simulink model "enginecontroller"  (R2015a)
settings: Solver=ode45  StartTime=0.0  StopTime=10.0  RelTol=1e-3
undefined symbols (not defined in the file): drive_block, drive_enginemodel, FuelConsTable, GasEmisTable, h, km, s, speed, torque
libraries: driveline x4, aerolibconvert2 x1, simulink x1
settings Model: Creator=Elena  LastModifiedBy=Elena

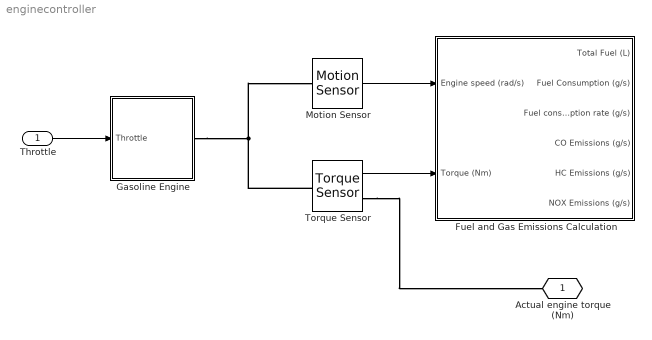
== system enginecontroller ==
  Throttle : Inport
  Fuel and Gas Emissions Calculation : Subsystem
  Gasoline Engine : Subsystem  AncestorBlock=driveline/Vehicle Components/Gasoline Engine  DialogController=PMDialogs.PMDefaultMaskDlg  LoadFcn=drive_block('LoadFcn');  StartFcn=drive_enginemodel('Start');  mask(Gasoline Engine){power_max=57000, speed_at_power_max=5000, speed_max=6000}
      mask prompts: power_max "Maximum power [W]:"; speed_at_power_max "Speed at maximum power [rpm]:"; speed_max "Maximum speed [rpm]:"
      mask help:
      | Simple gasoline fuel engine model with speed governor.  The throttle input signal lies between zero and one and specifies the torque demanded from the engine as a fraction of the maximum possible torque.  This signal also indirectly controls the engine speed.  The engine model does not include air-fuel combustion dynamics.
      |
      | If the throttle signal rises above one or falls below zero, the engine limits the signal to one or zero, respectively. If the engine speed rises above the maximum speed, the engine torque drops to zero.
      mask init:
      | drive_preinitmask();[speed,power,torque,p] = ...
      | 	drive_enginemodel('MaskGasoline');
      settings: CopyFcn=drive_block('CopyFcn');  DeleteFcn=drive_block('DeleteFcn');  ModelCloseFcn=drive_block('ModelCloseFcn');  PreSaveFcn=drive_block('PreSaveFcn');  PostSaveFcn=drive_block('PostSaveFcn');  PreCopyFcn=drive_block('PreCopyFcn');  PreDeleteFcn=drive_block('PreDeleteFcn');
      mask Help: web(drive_help);
      mask Display:
      | image(imread('engine.bmp'),'center')
      | plot(speed, torque/max(torque))
      | plot(speed, power/max(power))
      | port_label('input', 1, 'Throttle')
  Motion Sensor : driveline/Sensors & Actuators/Motion Sensor  Angle=off  x0=0  Velocity=on  Acceleration=off
  Torque Sensor : driveline/Sensors & Actuators/Torque Sensor
  Actual engine torque (Nm) : PMIOPort  Port=1  Side=Left
  wires:
  Throttle/1 -> Gasoline Engine/1(Throttle)
  Motion Sensor/1 -> Fuel and Gas Emissions Calculation/1(Engine speed (rad/s))
  Torque Sensor/1 -> Fuel and Gas Emissions Calculation/2(Torque (Nm))
  connections:
  Torque Sensor/RConn1 -- Actual engine torque (Nm)/RConn1
  Gasoline Engine/RConn1 -- Torque Sensor/LConn1 -- Motion Sensor/LConn1

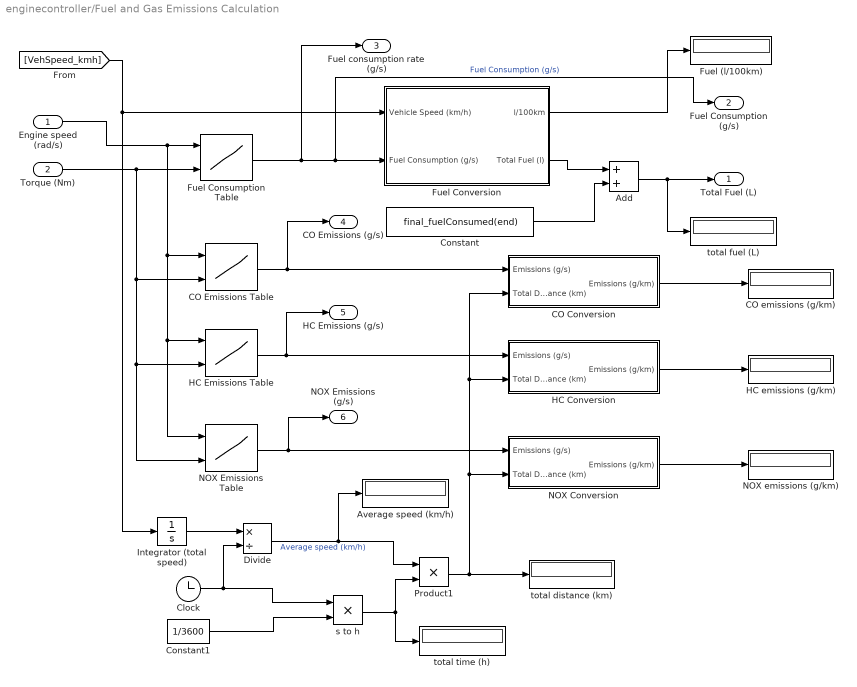
== system enginecontroller/Fuel and Gas Emissions Calculation ==
  Engine speed (rad/s) : Inport
  Torque (Nm) : Inport  Port=2
  Add : Sum
  Average speed (km/h) : Display
      settings: Decimation=100
  CO Conversion : Subsystem
  CO Emissions Table : Lookup2D  RowIndex=GasEmisTable.speed  ColumnIndex=GasEmisTable.torque  Table=GasEmisTable.lookupTableCO  LookUpMeth=Interpolation-Use End Values
  CO emissions (g/km) : Display
      settings: Decimation=100
  Clock : Clock
  Constant : Constant  Value=final_fuelConsumed(end)
  Constant1 : Constant  Value=1/3600
  Divide : Product  Inputs=*/
  Fuel Consumption Table : Lookup2D  RowIndex=FuelConsTable.speed  ColumnIndex=FuelConsTable.torque  Table=FuelConsTable.lookupTableFuel  LookUpMeth=Interpolation-Use End Values
  Fuel (l/100km) : Display
      settings: Decimation=100
  Fuel Conversion : Subsystem
  HC Conversion : Subsystem
  HC Emissions Table : Lookup2D  RowIndex=GasEmisTable.speed  ColumnIndex=GasEmisTable.torque  Table=GasEmisTable.lookupTableHC  LookUpMeth=Interpolation-Use End Values
  HC emissions (g/km) : Display
      settings: Decimation=100
  Integrator (total speed) : Integrator
  NOX Conversion : Subsystem
  NOX Emissions Table : Lookup2D  RowIndex=GasEmisTable.speed  ColumnIndex=GasEmisTable.torque  Table=GasEmisTable.lookupTableNOX  LookUpMeth=Interpolation-Use End Values
  NOX emissions (g/km) : Display
      settings: Decimation=100
  Product1 : Product
  s to h : Product
  total distance (km) : Display
      settings: Decimation=100
  total fuel (L) : Display
      settings: Decimation=100
  total time (h) : Display
      settings: Decimation=100
  Total Fuel (L) : Outport
  Fuel Consumption (g/s) : Outport  Port=2
  Fuel consumption rate (g/s) : Outport  Port=3
  CO Emissions (g/s) : Outport  Port=4
  HC Emissions (g/s) : Outport  Port=5
  NOX Emissions (g/s) : Outport  Port=6
  wires:
  Fuel Conversion/2(Total Fuel (l)) -> Add/1
  Fuel Consumption Table/1 -> Fuel consumption rate (g/s)/1, Fuel Consumption (g/s)/1, Fuel Conversion/2(Fuel Consumption (g/s))  "Fuel Consumption (g/s)"
  Fuel Conversion/1(l/100km) -> Fuel (l/100km)/1
  [VehSpeed_kmh] -> Fuel Conversion/1(Vehicle Speed (km/h)), Integrator (total speed)/1
  Torque (Nm)/1 -> Fuel Consumption Table/2, CO Emissions Table/2, HC Emissions Table/2, NOX Emissions Table/2
  Engine speed (rad/s)/1 -> Fuel Consumption Table/1, NOX Emissions Table/1, HC Emissions Table/1, CO Emissions Table/1
  HC Emissions Table/1 -> HC Conversion/1(Emissions (g/s)), HC Emissions (g/s)/1
  NOX Emissions Table/1 -> NOX Conversion/1(Emissions (g/s)), NOX Emissions (g/s)/1
  CO Emissions Table/1 -> CO Emissions (g/s)/1, CO Conversion/1(Emissions (g/s))
  Constant/1 -> Add/2
  Add/1 -> Total Fuel (L)/1, total fuel (L)/1
  Clock/1 -> s to h/1, Divide/2
  Constant1/1 -> s to h/2
  s to h/1 -> total time (h)/1, Product1/2
  Product1/1 -> NOX Conversion/2(Total Distance (km)), HC Conversion/2(Total Distance (km)), CO Conversion/2(Total Distance (km)), total distance (km)/1
  CO Conversion/1(Emissions (g/km)) -> CO emissions (g/km)/1
  HC Conversion/1(Emissions (g/km)) -> HC emissions (g/km)/1
  NOX Conversion/1(Emissions (g/km)) -> NOX emissions (g/km)/1
  Integrator (total speed)/1 -> Divide/1
  Divide/1 -> Average speed (km/h)/1, Product1/1  "Average speed (km/h)"

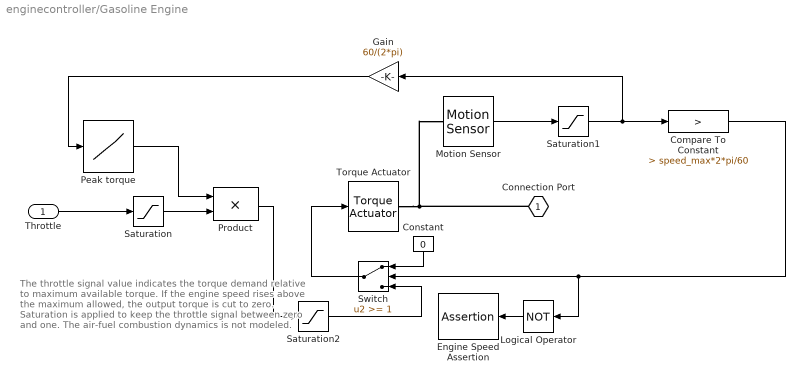
== system enginecontroller/Gasoline Engine ==
  note: The throttle signal value indicates the torque demand
      | relative to maximum available torque. If the engine
      | speed rises above the maximum allowed, the output
      | torque is cut to zero. Saturation is applied to keep the
      | throttle signal between zero and one.
      |
      | The air-fuel combustion dynamics is not modeled.
  Throttle : Inport
  Compare To Constant : simulink/Logic and Bit Operations/Compare To Constant  relop=>  const=speed_max*2*pi/60  OutDataTypeStr=uint8  ZeroCross=off
  Constant : Constant  Value=0
  Engine Speed Assertion : Assertion  AssertionFailFcn=disp('Engine speed (rpm) exceeded maximum speed during the simulation. Simulation results could be inaccurate or unpredictable.')  StopWhenAssertionFail=off
  Gain : Gain  Gain=60/(2*pi)
  Logical Operator : Logic  Operator=NOT  AllPortsSameDT=off  OutDataTypeStr=boolean
  Motion Sensor : driveline/Sensors & Actuators/Motion Sensor  Angle=off  x0=5  Velocity=on  Acceleration=off
  Peak torque : Lookup  InputValues=speed  Table=torque  SaturateOnIntegerOverflow=on
  Product : Product  SaturateOnIntegerOverflow=on  OutDataTypeStr=Inherit: Same as first input
  Saturation : Saturate  UpperLimit=1.0  LowerLimit=0.0
  Saturation1 : Saturate  UpperLimit=6000*pi/30  LowerLimit=0.0
  Saturation2 : Saturate  UpperLimit=136.0757  LowerLimit=0
  Switch : Switch  Threshold=1
  Torque Actuator : driveline/Sensors & Actuators/Torque Actuator
  Connection Port : PMIOPort  Port=1  Side=Right
  wires:
  Saturation/1 -> Product/2
  Throttle/1 -> Saturation/1
  Constant/1 -> Switch/1
  Compare To Constant/1 -> Switch/2, Logical Operator/1
  Product/1 -> Saturation2/1
  Motion Sensor/1 -> Saturation1/1
  Peak torque/1 -> Product/1
  Logical Operator/1 -> Engine Speed Assertion/1
  Saturation1/1 -> Gain/1, Compare To Constant/1
  Switch/1 -> Torque Actuator/1
  Gain/1 -> Peak torque/1
  Saturation2/1 -> Switch/3
  connections:
  Connection Port/RConn1 -- Torque Actuator/RConn1 -- Motion Sensor/LConn1

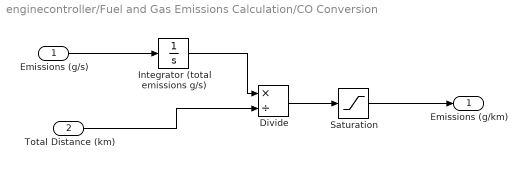
== system enginecontroller/Fuel and Gas Emissions Calculation/CO Conversion ==
  Emissions (g/s) : Inport
  Total Distance (km) : Inport  Port=2
  Divide : Product  Inputs=*/
  Integrator (total emissions g/s) : Integrator  InitialCondition=eps
  Saturation : Saturate  UpperLimit=Inf  LowerLimit=0
  Emissions (g/km) : Outport
  wires:
  Divide/1 -> Saturation/1
  Emissions (g/s)/1 -> Integrator (total emissions g/s)/1
  Integrator (total emissions g/s)/1 -> Divide/1
  Total Distance (km)/1 -> Divide/2
  Saturation/1 -> Emissions (g/km)/1

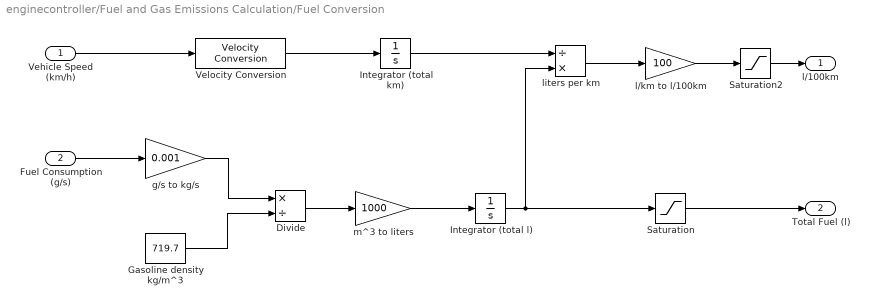
== system enginecontroller/Fuel and Gas Emissions Calculation/Fuel Conversion ==
  Vehicle Speed (km/h) : Inport
  Fuel Consumption (g/s) : Inport  Port=2
  Divide : Product  Inputs=*/
  Gasoline density kg/m^3 : Constant  Value=719.7
  Integrator (total km) : Integrator  InitialCondition=eps
  Integrator (total l) : Integrator  InitialCondition=eps
  Saturation : Saturate  UpperLimit=Inf  LowerLimit=0
  Saturation2 : Saturate  UpperLimit=15  LowerLimit=0
  Velocity Conversion : aerolibconvert2/Velocity Conversion  IU=km/h  OU=km/s
  g/s to kg/s : Gain  Gain=0.001
  l/km to l/100km : Gain  Gain=100
  liters per km : Product  Inputs=/*
  m^3 to liters : Gain  Gain=1000
  l/100km : Outport
  Total Fuel (l) : Outport  Port=2
  wires:
  Vehicle Speed (km/h)/1 -> Velocity Conversion/1
  Velocity Conversion/1 -> Integrator (total km)/1
  Fuel Consumption (g/s)/1 -> g/s to kg/s/1
  g/s to kg/s/1 -> Divide/1
  Gasoline density kg/m^3/1 -> Divide/2
  Divide/1 -> m^3 to liters/1
  m^3 to liters/1 -> Integrator (total l)/1
  Integrator (total km)/1 -> liters per km/1
  Integrator (total l)/1 -> Saturation/1, liters per km/2
  liters per km/1 -> l/km to l/100km/1
  l/km to l/100km/1 -> Saturation2/1
  Saturation/1 -> Total Fuel (l)/1
  Saturation2/1 -> l/100km/1

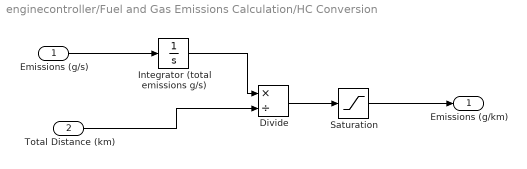
== system enginecontroller/Fuel and Gas Emissions Calculation/HC Conversion ==
  Emissions (g/s) : Inport
  Total Distance (km) : Inport  Port=2
  Divide : Product  Inputs=*/
  Integrator (total emissions g/s) : Integrator  InitialCondition=eps
  Saturation : Saturate  UpperLimit=Inf  LowerLimit=0
  Emissions (g/km) : Outport
  wires:
  Divide/1 -> Saturation/1
  Emissions (g/s)/1 -> Integrator (total emissions g/s)/1
  Integrator (total emissions g/s)/1 -> Divide/1
  Total Distance (km)/1 -> Divide/2
  Saturation/1 -> Emissions (g/km)/1

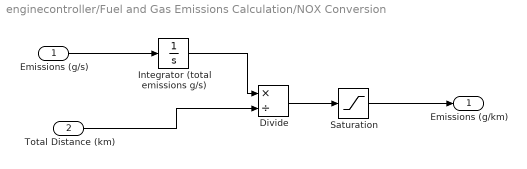
== system enginecontroller/Fuel and Gas Emissions Calculation/NOX Conversion ==
  Emissions (g/s) : Inport
  Total Distance (km) : Inport  Port=2
  Divide : Product  Inputs=*/
  Integrator (total emissions g/s) : Integrator  InitialCondition=eps
  Saturation : Saturate  UpperLimit=Inf  LowerLimit=0
  Emissions (g/km) : Outport
  wires:
  Divide/1 -> Saturation/1
  Emissions (g/s)/1 -> Integrator (total emissions g/s)/1
  Integrator (total emissions g/s)/1 -> Divide/1
  Total Distance (km)/1 -> Divide/2
  Saturation/1 -> Emissions (g/km)/1
